simulink model "modell"  (Simulink 7.6)
settings: Solver=ode45  StartTime=0.0  StopTime=10.0  RelTol=1e-3
undefined symbols (not defined in the file or in its folder): x10, x20
settings Model: Creator=Attila  LastModifiedBy=Attila

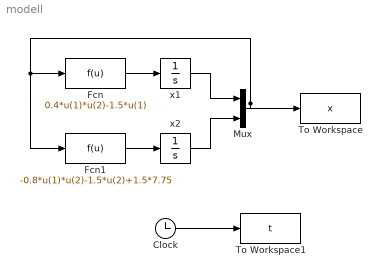
== system modell ==
  Clock : Clock
      settings: Decimation=10
  Fcn : Fcn  Expr=0.4*u(1)*u(2)-1.5*u(1)
  Fcn1 : Fcn  Expr=-0.8*u(1)*u(2)-1.5*u(2)+1.5*7.75
  Mux : Mux  Inputs=2
  To Workspace : ToWorkspace  VariableName=x  SampleTime=-1  SaveFormat=Array
  To Workspace1 : ToWorkspace  VariableName=t  SampleTime=-1  SaveFormat=Array
  x1 : Integrator  InitialCondition=x10
  x2 : Integrator  InitialCondition=x20
  wires:
  x1/1 -> Mux/1
  Fcn/1 -> x1/1
  Fcn1/1 -> x2/1
  Mux/1 -> Fcn1/1, Fcn/1, To Workspace/1
  Clock/1 -> To Workspace1/1
  x2/1 -> Mux/2
